simulink model "blockdemo"  (Simulink 6.4)
settings: Solver=ode45  StartTime=0.0  StopTime=400  RelTol=1e-3
InitFcn:
  | %% DSPBuilder Start
  | alt_dspbuilder_update_model(bdroot)
  | %% DSPBuilder End
libraries: allblocks_alteradspbuilder2 x7
settings Model: Creator=cpurcell  LastModifiedBy=lkong
settings OptimizationCC: BlockReduction=off  BooleanDataType=off  InlineInvariantSignals=on
settings DebuggingCC: SolverPrmCheckMsg=none
settings HardwareCC: TargetUnknown=on

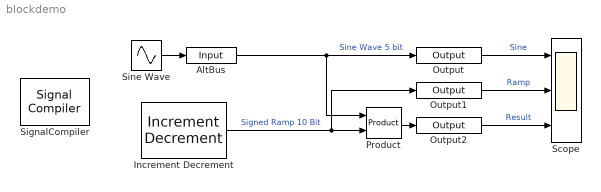
== system blockdemo ==
  AltBus : allblocks_alteradspbuilder2/Input  iofile=D:\wsTrunk\workspace\Documentation\DesignExamples\Tutorials\UnitBlocks\Arithmetic\Product\tb_blockdemo\blockdemo_AltBus.salt  BusType=Signed Integer  bwl=5  bwr=4  SpecifyClock=off  PORTTYPE=Input  externalType=Inferred  allowFloatingPointOverride=on  logOutputs=off
  Increment Decrement : allblocks_alteradspbuilder2/Increment Decrement  BusType=Signed Integer  bwl=10  bwr=0  SpecifyClock=off  clr_value=0  direction=Increment  phase_selection=1  use_ena=off  use_sclr=off  pipeline_display=1
  Output : allblocks_alteradspbuilder2/Output  iofile=D:\wsTrunk\workspace\Documentation\DesignExamples\Tutorials\UnitBlocks\Arithmetic\Product\tb_blockdemo\blockdemo_Output.capture  BusType=Signed Integer  bwl=5  bwr=0  externalType=Inferred  PORTTYPE=Output  allowFloatingPointOverride=on  logOutputs=off
  Output1 : allblocks_alteradspbuilder2/Output  iofile=D:\wsTrunk\workspace\Documentation\DesignExamples\Tutorials\UnitBlocks\Arithmetic\Product\tb_blockdemo\blockdemo_Output1.capture  BusType=Signed Integer  bwl=10  bwr=0  externalType=Inferred  PORTTYPE=Output  allowFloatingPointOverride=on  logOutputs=off
  Output2 : allblocks_alteradspbuilder2/Output  iofile=D:\wsTrunk\workspace\Documentation\DesignExamples\Tutorials\UnitBlocks\Arithmetic\Product\tb_blockdemo\blockdemo_Output2.capture  BusType=Signed Integer  bwl=50  bwr=0  externalType=Inferred  PORTTYPE=Output  allowFloatingPointOverride=on  logOutputs=off
  Product : allblocks_alteradspbuilder2/Product  BusType=Inferred  bwl=8  bwr=0  pipeline=3  pipeline_display=3  phase_selection=1  use_ena=off  use_aclr=off  UseLPM=off  UseDedicatedCircuitry=off  allowFloatingPointOverride=on  logOutputs=off  logFile=D:\wsTrunk\workspace\Documentation\DesignExamples\Tutorials\UnitBlocks\Arithmetic\Product\tb_blockdemo\blockdemo_Product.fixedpointlog
  Scope : Scope  NumInputPorts=3
      settings: YMin=-20~0~-5000  YMax=20~400~5000
  SignalCompiler : allblocks_alteradspbuilder2/Signal Compiler  DeviceFamily=Stratix IV  DeviceName=AUTO  EnableSignalTap=off  SignalTapDepth=128  UseBoardBlock=off  StpUseDefaultClock=on  StpClock=Clock  ExportDir=D:\MATLAB\R2006a\work
  Sine Wave : Sin  Amplitude=15  Frequency=0.2  Phase=2  SampleTime=0
  wires:
  Sine Wave/1 -> AltBus/1
  Product/1 -> Output2/1
  Increment Decrement/1 -> Product/2, Output1/1  "Signed Ramp 10 Bit"
  AltBus/1 -> Product/1, Output/1  "Sine Wave 5 bit"
  Output/1 -> Scope/1  "Sine"
  Output1/1 -> Scope/2  "Ramp"
  Output2/1 -> Scope/3  "Result"
